simulink subsystem "Motor"  (R2024a)
settings: Solver=VariableStepAuto  StartTime=0.0  StopTime=10.0  RelTol=1e-3
undefined symbols (not defined in the file): I_DC_load, I_RMS, rpm_grid, throttle_grid, TORQUE, V_DC_load, V_RMS
settings Model: Creator=User  LastModifiedBy=User

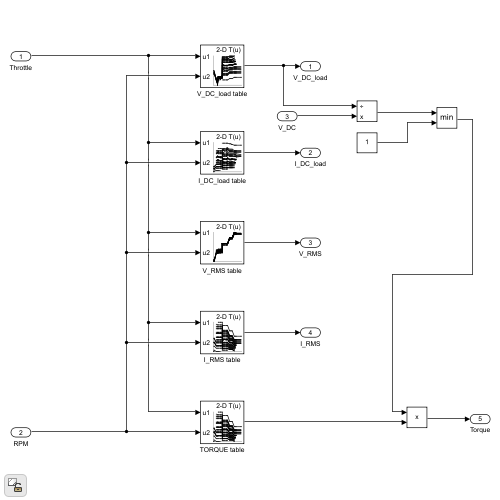
[thumbnail: Simulink's stored preview of the top-level diagram]
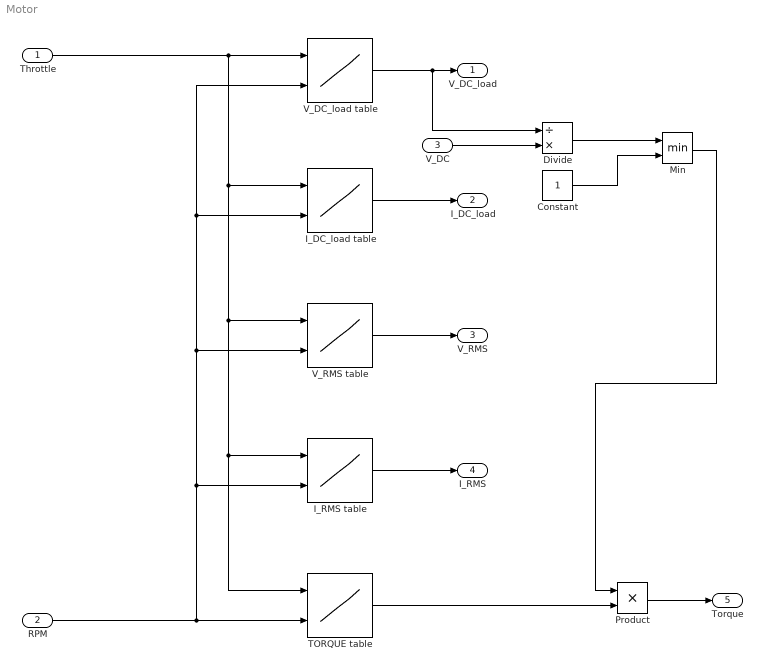
== system Motor ==
  Throttle : Inport
  RPM : Inport  Port=2
  V_DC : Inport  Port=3
  Constant : Constant
  Divide : Product  Inputs=/*
  I_DC_load table : Lookup_n-D  BreakpointsForDimension1=throttle_grid  BreakpointsForDimension2=rpm_grid  Table=I_DC_load  InternalRulePriority=Speed  RndMeth=Simplest
      settings: InputPortMap=u0,u1
  I_RMS table : Lookup_n-D  BreakpointsForDimension1=throttle_grid  BreakpointsForDimension2=rpm_grid  Table=I_RMS  InternalRulePriority=Speed  RndMeth=Simplest
      settings: InputPortMap=u0,u1
  Min : MinMax  Inputs=2
  Product : Product
  TORQUE table : Lookup_n-D  BreakpointsForDimension1=throttle_grid  BreakpointsForDimension2=rpm_grid  Table=TORQUE  InternalRulePriority=Speed  RndMeth=Simplest
      settings: InputPortMap=u0,u1
  V_DC_load table : Lookup_n-D  BreakpointsForDimension1=throttle_grid  BreakpointsForDimension2=rpm_grid  Table=V_DC_load  InterpMethod=Linear Lagrange  InternalRulePriority=Speed  RndMeth=Simplest
      settings: InputPortMap=u0,u1
  V_RMS table : Lookup_n-D  BreakpointsForDimension1=throttle_grid  BreakpointsForDimension2=rpm_grid  Table=V_RMS  InternalRulePriority=Speed  RndMeth=Simplest
      settings: InputPortMap=u0,u1
  V_DC_load : Outport
  I_DC_load : Outport  Port=2
  V_RMS : Outport  Port=3
  I_RMS : Outport  Port=4
  Torque : Outport  Port=5
  wires:
  Throttle/1 -> TORQUE table/1, I_RMS table/1, V_RMS table/1, I_DC_load table/1, V_DC_load table/1
  RPM/1 -> I_RMS table/2, V_RMS table/2, I_DC_load table/2, V_DC_load table/2, TORQUE table/2
  I_DC_load table/1 -> I_DC_load/1
  V_RMS table/1 -> V_RMS/1
  I_RMS table/1 -> I_RMS/1
  V_DC_load table/1 -> Divide/1, V_DC_load/1
  V_DC/1 -> Divide/2
  Divide/1 -> Min/1
  Constant/1 -> Min/2
  TORQUE table/1 -> Product/2
  Product/1 -> Torque/1
  Min/1 -> Product/1
